simulink model "dual_track_model"  (R2018b)
settings: Solver=VariableStepAuto  StartTime=0.0  StopTime=50  RelTol=1e-3
libraries: simulink x1, autolibshared x1
settings Model: Creator=rhs2rng  LastModifiedBy=rhs2rng

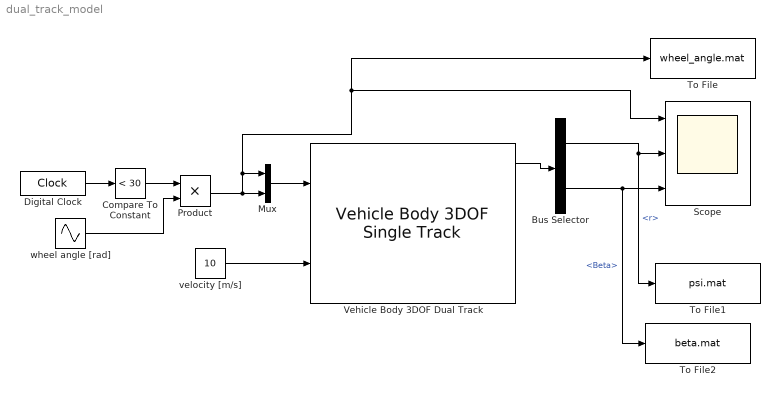
== system dual_track_model ==
  Bus Selector : BusSelector  OutputSignals=BdyFrm.Cg.AngVel.r,BdyFrm.Cg.Ang.Beta
  Compare To Constant : simulink/Logic and Bit Operations/Compare To Constant  relop=<  const=30  OutDataTypeStr=boolean
  Digital Clock : DigitalClock
  Mux : Mux  Inputs=2
  Product : Product
  Scope : Scope  NumInputPorts=3
  To File : ToFile  Filename=wheel_angle.mat  SampleTime=0.01
  To File1 : ToFile  Filename=psi.mat  SampleTime=0.01
  To File2 : ToFile  Filename=beta.mat  SampleTime=0.01
  Vehicle Body 3DOF Dual Track : autolibshared/Vehicle Body 3DOF Single Track  trackMode=Dual  inputMode=External longitudinal velocity  frontSteerMode=on  rearSteerMode=off  windMode=off  muMode=off  extFMode=off  extMMode=off  aMode=2  NF=2  NR=2  m=2000  a=1.4  b=1.6  h=0.35  X_o=0  xdot_o=0  CalphaMode=off  sigmaMode=on  d=0  w=[1.4,1.4]  Cy_f=12e3  Cy_r=11e3  sigma_f=.1  sigma_r=.1  alpha_f_brk=[-.1 .1]  Cy_f_data=[-9e3 9e3]  alpha_r_brk=[-.1 .1]  Cy_r_data=[-9e3 9e3]  Y_o=0  ydot_o=0  Izz=4000  psi_o=0  r_o=0  Af=2  Cd=.3  Cl=.1  Cpm=.1  beta_w=[0:0.01:0.3]  Cs=[0:0.03:0.9]  Cym=[0:0.01:0.3]  Pabs=101325  Tair=273  g=9.81  mu=1  xdot_tol=.01  Fznom=5000  Fxtire_sat=7e4  Fytire_sat=7e4  longOff=0  latOff=0  vertOff=0
      settings: SourceProductName=Powertrain Blockset  SourceProductBaseCode=PW
  velocity [m/s] : Constant  Value=10
  wheel angle [rad] : Sin  SineType=Sample based  Amplitude=0.4  Frequency=0.5  Samples=1000  SampleTime=0.01
  wires:
  velocity [m/s]/1 -> Vehicle Body 3DOF Dual Track/2
  Vehicle Body 3DOF Dual Track/1 -> Bus Selector/1
  Bus Selector/1 -> To File1/1, Scope/2  "<r>"
  Bus Selector/2 -> To File2/1, Scope/3  "<Beta>"
  Digital Clock/1 -> Compare To Constant/1
  Compare To Constant/1 -> Product/1
  wheel angle [rad]/1 -> Product/2
  Product/1 -> Scope/1, To File/1, Mux/1, Mux/2
  Mux/1 -> Vehicle Body 3DOF Dual Track/1
